simulink model "TransientPEMFC"  (R2025a)
settings: Solver=VariableStepAuto  StartTime=0.0  StopTime=10.0  RelTol=1e-3
InitFcn:
  | pyenv_setup(); create_buses(5);
settings Model: Creator=paffonsonobrega  LastModifiedBy=paffonsonobrega

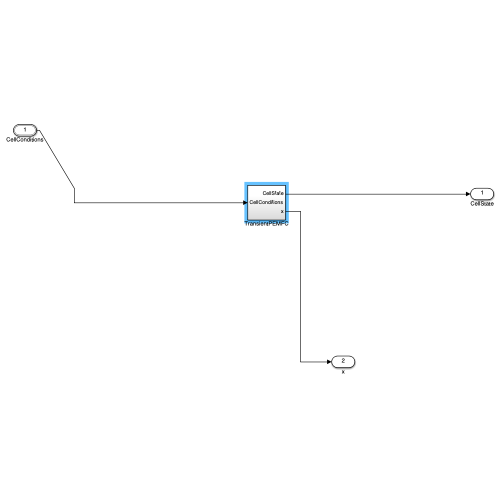
[thumbnail: Simulink's stored preview of the top-level diagram]
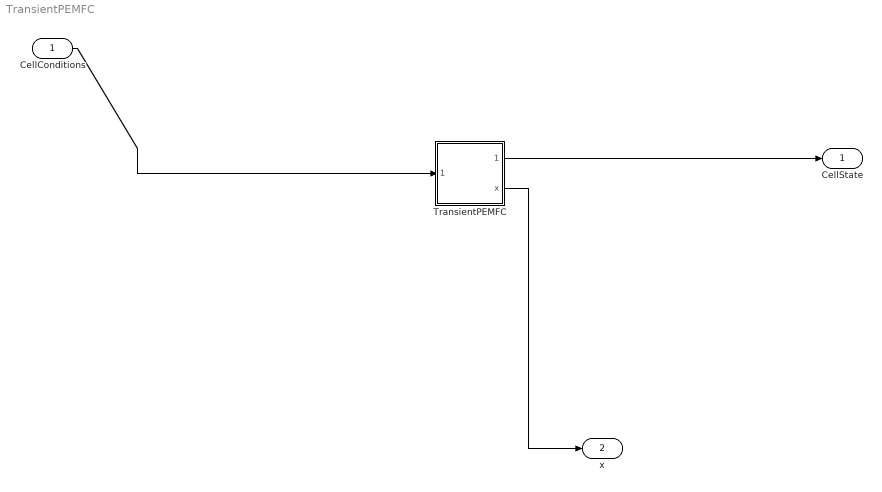
== system TransientPEMFC ==
  CellConditions : Inport  OutDataTypeStr=Bus: CellConditionsBus
  TransientPEMFC : Subsystem  mask(TransientPEMFC){n_memb_mesh=5, cellBuilderExpr='marapendi.interop.simulink_bridge.build_default_cell', x0=[0.978373133858763 0.811460140922502 0.856472884136313 0.903807555680236 0.953582665236504 1.00592271864168]}
      mask prompts: n_memb_mesh "Membrane mesh nodes (n_memb_mesh)"; cellBuilderExpr "Python cell-builder function (dotted path)"; x0 "Initial ODE state x0 (1 x n_memb_mesh+1)"
      mask help:
      | Encapsulates marapendi.models.base.transient.TransientModel
      | (coupled MEA temperature / membrane water-content ODE) via a Python-calling S-Function.
      | Edit the physics in the marapendi Python package; this block always calls the live model.
  CellState : Outport
  x : Outport  Port=2
  wires:
  CellConditions/1 -> TransientPEMFC/1(CellConditions)
  TransientPEMFC/1(CellState) -> CellState/1
  TransientPEMFC/2(x) -> x/1

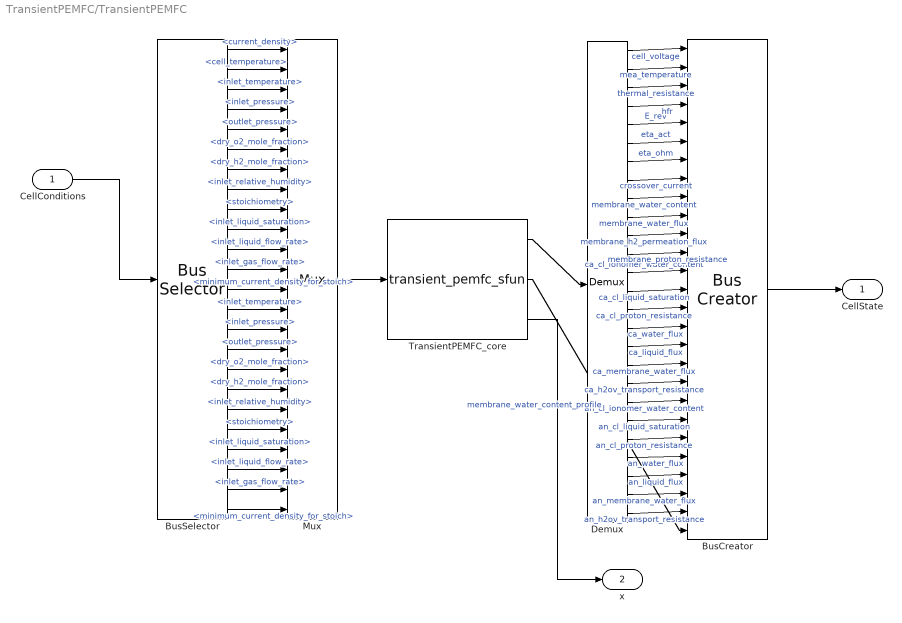
== system TransientPEMFC/TransientPEMFC ==
  CellConditions : Inport  OutDataTypeStr=Bus: CellConditionsBus
  BusCreator : BusCreator  Inputs=27  OutDataTypeStr=Bus: CellStateBus  NonVirtualBus=on
  BusSelector : BusSelector  OutputSignals=current_density,cell_temperature,ca.inlet_temperature,ca.inlet_pressure,ca.outlet_pressure,ca.dry_o2_mole_fraction,ca.dry_h2_mole_fraction,ca.inlet_relative_humidity,ca.stoichiometry,ca.inlet_liquid_saturation,ca.inlet_liquid_flow_rate,ca.inlet_gas_flow_rate,ca.minimum_current_density_for_stoich,an.inlet_temperature,an.inlet_pressure,an.outlet_pressure,an.dry_o2_mole_fraction,an.dry_h2_mole_fraction,an.inlet_relative_humidity,an.stoichiometry,an.inlet_liquid_saturation,an.inlet_liquid_flow_rate,an.inlet_gas_flow_rate,an.minimum_current_density_for_stoich
  Demux : Demux  Outputs=26
  Mux : Mux  Inputs=24
  TransientPEMFC_core : M-S-Function  FunctionName=transient_pemfc_sfun  Parameters=n_memb_mesh, cellBuilderExpr, x0
  CellState : Outport
  x : Outport  Port=2
  wires:
  Mux/1 -> TransientPEMFC_core/1
  BusSelector/2 -> Mux/2  "<cell_temperature>"
  BusSelector/4 -> Mux/4  "<inlet_pressure>"
  BusSelector/3 -> Mux/3  "<inlet_temperature>"
  BusSelector/5 -> Mux/5  "<outlet_pressure>"
  Demux/5 -> BusCreator/5  "E_rev"
  BusSelector/11 -> Mux/11  "<inlet_liquid_flow_rate>"
  BusSelector/12 -> Mux/12  "<inlet_gas_flow_rate>"
  BusSelector/15 -> Mux/15  "<inlet_pressure>"
  BusSelector/21 -> Mux/21  "<inlet_liquid_saturation>"
  Demux/13 -> BusCreator/13  "ca_cl_ionomer_water_content"
  TransientPEMFC_core/1 -> Demux/1
  BusSelector/1 -> Mux/1  "<current_density>"
  BusSelector/22 -> Mux/22  "<inlet_liquid_flow_rate>"
  BusSelector/7 -> Mux/7  "<dry_h2_mole_fraction>"
  BusSelector/6 -> Mux/6  "<dry_o2_mole_fraction>"
  Demux/24 -> BusCreator/24  "an_liquid_flux"
  Demux/22 -> BusCreator/22  "an_cl_proton_resistance"
  Demux/2 -> BusCreator/2  "mea_temperature"
  BusSelector/17 -> Mux/17  "<dry_o2_mole_fraction>"
  Demux/11 -> BusCreator/11  "membrane_h2_permeation_flux"
  Demux/3 -> BusCreator/3  "thermal_resistance"
  Demux/1 -> BusCreator/1  "cell_voltage"
  Demux/26 -> BusCreator/26  "an_h2ov_transport_resistance"
  BusCreator/1 -> CellState/1
  CellConditions/1 -> BusSelector/1
  Demux/23 -> BusCreator/23  "an_water_flux"
  Demux/20 -> BusCreator/20  "an_cl_ionomer_water_content"
  Demux/15 -> BusCreator/15  "ca_cl_proton_resistance"
  TransientPEMFC_core/2 -> BusCreator/27  "membrane_water_content_profile"
  BusSelector/19 -> Mux/19  "<inlet_relative_humidity>"
  BusSelector/9 -> Mux/9  "<stoichiometry>"
  BusSelector/16 -> Mux/16  "<outlet_pressure>"
  Demux/4 -> BusCreator/4  "hfr"
  Demux/8 -> BusCreator/8  "crossover_current"
  Demux/10 -> BusCreator/10  "membrane_water_flux"
  BusSelector/24 -> Mux/24  "<minimum_current_density_for_stoich>"
  Demux/14 -> BusCreator/14  "ca_cl_liquid_saturation"
  Demux/6 -> BusCreator/6  "eta_act"
  BusSelector/20 -> Mux/20  "<stoichiometry>"
  BusSelector/14 -> Mux/14  "<inlet_temperature>"
  TransientPEMFC_core/3 -> x/1
  Demux/18 -> BusCreator/18  "ca_membrane_water_flux"
  BusSelector/23 -> Mux/23  "<inlet_gas_flow_rate>"
  BusSelector/13 -> Mux/13  "<minimum_current_density_for_stoich>"
  BusSelector/10 -> Mux/10  "<inlet_liquid_saturation>"
  Demux/21 -> BusCreator/21  "an_cl_liquid_saturation"
  Demux/12 -> BusCreator/12  "membrane_proton_resistance"
  Demux/16 -> BusCreator/16  "ca_water_flux"
  Demux/19 -> BusCreator/19  "ca_h2ov_transport_resistance"
  BusSelector/8 -> Mux/8  "<inlet_relative_humidity>"
  Demux/17 -> BusCreator/17  "ca_liquid_flux"
  Demux/7 -> BusCreator/7  "eta_ohm"
  BusSelector/18 -> Mux/18  "<dry_h2_mole_fraction>"
  Demux/25 -> BusCreator/25  "an_membrane_water_flux"
  Demux/9 -> BusCreator/9  "membrane_water_content"
